simulink model "simulink_test"  (R2021a)
settings: Solver=VariableStepAuto  StartTime=0.0  StopTime=10.0  RelTol=1e-3
undefined symbols (not defined in the file or in its folder): Bl, Cm, Le, Mm, Re, Rm, s
settings Model: Creator=padlewsk  LastModifiedBy=padlewsk

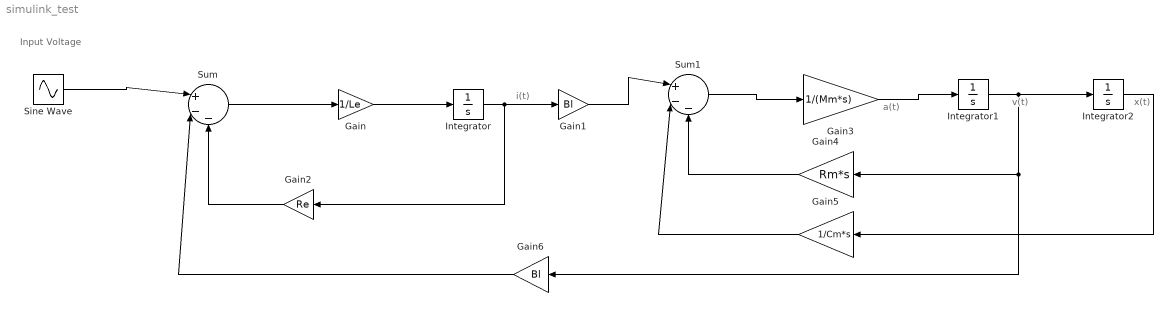
== system simulink_test ==
  note: Input Voltage
  note: i(t)
  note: a(t)
  note: v(t)
  note: x(t)
  Gain : Gain  Gain=1/Le
  Gain1 : Gain  Gain=Bl
  Gain2 : Gain  Gain=Re
  Gain3 : Gain  Gain=1/(Mm*s)
  Gain4 : Gain  Gain=Rm*s
  Gain5 : Gain  Gain=1/Cm*s
  Gain6 : Gain  Gain=Bl
  Integrator : Integrator
  Integrator1 : Integrator
  Integrator2 : Integrator
  Sine Wave : Sin  SampleTime=0
  Sum : Sum  Inputs=|+--
  Sum1 : Sum  Inputs=|+--
  wires:
  Sine Wave/1 -> Sum/1
  Sum/1 -> Gain/1
  Gain/1 -> Integrator/1
  Integrator/1 -> Gain2/1, Gain1/1
  Gain2/1 -> Sum/3
  Gain1/1 -> Sum1/1
  Sum1/1 -> Gain3/1
  Gain3/1 -> Integrator1/1
  Integrator1/1 -> Integrator2/1, Gain6/1, Gain4/1
  Integrator2/1 -> Gain5/1
  Gain6/1 -> Sum/2
  Gain5/1 -> Sum1/2
  Gain4/1 -> Sum1/3
